simulink model "ac_levitation"  (R2018b)
settings: Solver=FixedStepDiscrete  StartTime=0.0  StopTime=inf  FixedStep=10  RelTol=1e-3  EnableMultiTasking=on
settings Model: SimulationMode=external  Creator=Josef  LastModifiedBy=Josef
settings SolverCC: PositivePriorityOrder=on
settings OptimizationCC: PassReuseOutputArgsThreshold=0  MaxStackSize=64
settings DebuggingCC: ParameterTunabilityLossMsg=error
settings HardwareCC: ProdBitPerPointer=32  ProdBitPerSizeT=32  ProdBitPerPtrDiffT=32  ProdLargestAtomicInteger=Long  ProdLargestAtomicFloat=Double  ProdWordSize=32  ProdHWDeviceType=ARM Compatible->ARM Cortex  UseEmbeddedCoderFeatures=off
settings SFSimCC: SimUseLocalCustomCode=off  MATLABDynamicMemAlloc=off
settings RTWCC: SystemTargetFile=ert.tlc  HardwareBoard=Raspberry Pi  TLCOptions="-aInlineSetEventsForThisBaseRateFcn=TLC_FALSE -aSuppressMultiTaskScheduler=TLC_FALSE  -aRateBasedStepFcn=0"  TemplateMakefile=ert_default_tmf  GenerateReport=on  RTWUseLocalCustomCode=off  Toolchain=GNU GCC Raspberry Pi  TargetLang=C++
settings CodeAppCC: ForceParamTrailComments=on  OperatorAnnotations=on
settings ERTTargetCC: TargetLangStandard=C++03 (ISO)  ERTCustomFileBanners=off  SupportContinuousTime=on  SupportNonInlinedSFcns=on  RemoveResetFunc=off  SupportVariableSizeSignals=on  ModelStepFunctionPrototypeControlCompliant=off

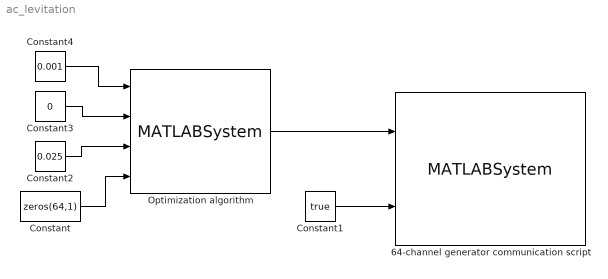
== system ac_levitation ==
  64-channel generator communication script : MATLABSystem  System=NewGenerator  Port=/dev/ttyUSB0  Baud=230400
      mask Type: NewGenerator
      mask Display:
      | disp(['64 phase generator' char(10) ' Port: /dev/ttyUSB0' char(10) ' Baudrate: 230400']);
      | port_label('input',1,'phases');
      | port_label('input',2,'On/Off');
  Constant : Constant  Value=zeros(64,1)
  Constant1 : Constant  Value=true
  Constant2 : Constant  Value=0.025
  Constant3 : Constant  Value=0
  Constant4 : Constant  Value=0.001
  Optimization algorithm : MATLABSystem  System=Levitation  cp=2350  rhop=29.36  rp=1e-3  c0=343  rho0=1.2  wp=0.1  wx=1500  wy=1500  wz=100
      mask Type: Levitation
      mask Display:
      | disp(['Levitation' char(10) 'optimization']);
      | port_label('input',1,'x');
      | port_label('input',2,'y');
      | port_label('input',3,'z');
      | port_label('input',4,'Initial condition');
      | port_label('output',1,'Phases');
  wires:
  Constant1/1 -> 64-channel generator communication script/2
  Optimization algorithm/1 -> 64-channel generator communication script/1
  Constant/1 -> Optimization algorithm/4
  Constant2/1 -> Optimization algorithm/3
  Constant3/1 -> Optimization algorithm/2
  Constant4/1 -> Optimization algorithm/1
